simulink model "FullEKF_2007a"  (Simulink 6.6)
settings: Solver=FixedStepDiscrete  StartTime=0.0  StopTime=300  FixedStep=0.01  RelTol=1e-3
values from neighbouring files (symbols this model uses):
  initP = diag([1e-3 1e-3 1e-3 1e-6 1e-6 1e-6 1 1 1 5e-6 5e-6 5e-6 1e-8 1e-8 1e-8])    [FullEKF_init.m.m]
undefined symbols (not defined in the file or in its folder): DiscIntNeverNeededParam, gcbh, hwbcalib_subsystem
libraries: simulink x6, dspmtrx3 x4, dspinverses x1
(part 1 of 7)
settings Model: Creator=Markéta  LastModifiedBy=Markéta
settings OptimizationCC: InitFltsAndDblsToZero=off
settings DebuggingCC: StrictBusMsg=ErrorLevel1
settings HardwareCC: TargetHWDeviceType=32-bit Generic

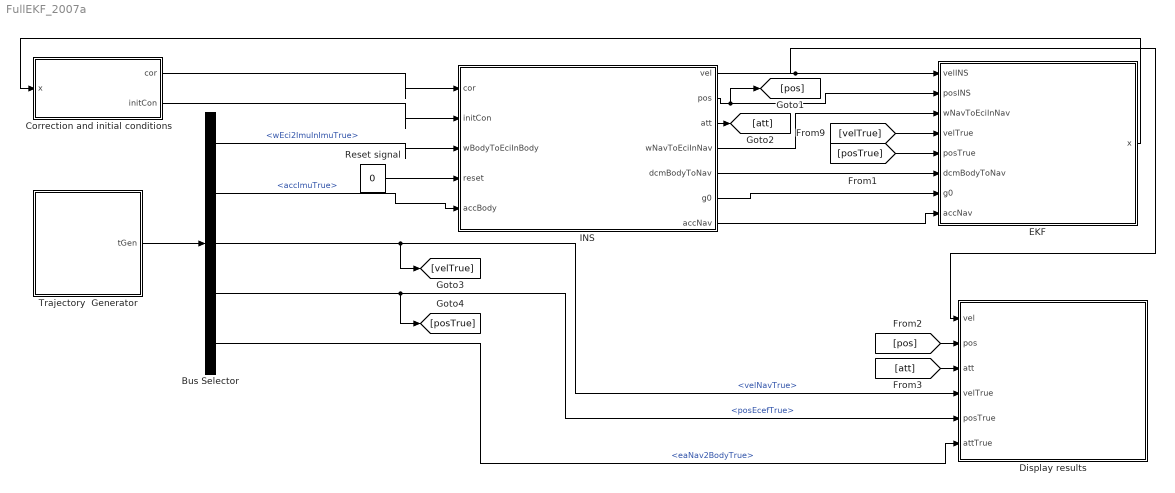
== system FullEKF_2007a ==
  Bus Selector : BusSelector  OutputSignals=state.wEci2ImuInImuTrue,state.accImuTrue,state.velNavTrue,state.posEcefTrue,state.eaNav2BodyTrue
  Correction and initial conditions : Subsystem
  Display results : Subsystem
  EKF : Subsystem
  INS : Subsystem
  Reset signal : Constant  Value=0  OutDataType=fixdt(1,16,0)  OutScaling=[]  SampleTime=0.01
  Trajectory  Generator : Subsystem
      settings: CopyFcn=|
      | if exist('gnlib_subsystem')
      |    gnlib_subsystem(gcbh, 'title')
      | end
      settings: NameChangeFcn=|
      | if exist('gnlib_subsystem')
      |    gnlib_subsystem(gcbh, 'title')
      | end
  wires:
  Trajectory  Generator/1(tGen) -> Bus Selector/1
  Bus Selector/2 -> INS/5(accBody)  "<accImuTrue>"
  Bus Selector/1 -> INS/3(wBodyToEciInBody)  "<wEci2ImuInImuTrue>"
  Correction and initial conditions/1(cor) -> INS/1(cor)
  Correction and initial conditions/2(initCon) -> INS/2(initCon)
  INS/1(vel) -> EKF/1(velINS), Display results/1(vel)
  INS/2(pos) -> EKF/2(posINS), [pos]
  Reset signal/1 -> INS/4(reset)
  EKF/1(x) -> Correction and initial conditions/1(x)
  INS/6(g0) -> EKF/7(g0)
  INS/4(wNavToEciInNav) -> EKF/3(wNavToEciInNav)
  INS/5(dcmBodyToNav) -> EKF/6(dcmBodyToNav)
  INS/7(accNav) -> EKF/8(accNav)
  Bus Selector/5 -> Display results/6(attTrue)  "<eaNav2BodyTrue>"
  Bus Selector/3 -> Display results/4(velTrue), [velTrue]  "<velNavTrue>"
  Bus Selector/4 -> Display results/5(posTrue), [posTrue]  "<posEcefTrue>"
  [posTrue] -> EKF/5(posTrue)
  [velTrue] -> EKF/4(velTrue)
  INS/3(att) -> [att]
  [att] -> Display results/3(att)
  [pos] -> Display results/2(pos)

== system FullEKF_2007a/Correction and initial conditions ==
  note: velInitCon
  note: posInitCon
  note: attInitCon
  note: corToAtt
  note: corToPos
  x : Inport  SampleTime=0.01  OutDataType=fixdt(1,16,0)  OutScaling=[]
  Bus Creator : BusCreator  Inputs=5
  Bus Creator1 : BusCreator  Inputs=3
  Demux : Demux  Outputs=5
  Demux2 : Demux  Outputs=3
  Gain{1..3,5} (4 alike) : Gain  ParameterDataType=fixdt(1,16,0)  ParameterScaling=[]  OutDataType=fixdt(1,16,0)  OutScaling=[]
  Gain4 : Gain  Gain=0  ParameterDataType=fixdt(1,16,0)  ParameterScaling=[]  OutDataType=fixdt(1,16,0)  OutScaling=[]
  accBias : Scope
      settings: TimeRange=50  YMin=-2.9e-014  YMax=-1.4e-014  SaveName=ScopeData4
  biasAcumulator1 : Subsystem
      settings: CopyFcn=|
      | if exist('gnlib_subsystem')
      |    gnlib_subsystem(gcbh, 'title')
      | end
      settings: NameChangeFcn=|
      | if exist('gnlib_subsystem')
      |    gnlib_subsystem(gcbh, 'title')
      | end
  biasAcumulator2 : Subsystem
      settings: CopyFcn=|
      | if exist('gnlib_subsystem')
      |    gnlib_subsystem(gcbh, 'title')
      | end
      settings: NameChangeFcn=|
      | if exist('gnlib_subsystem')
      |    gnlib_subsystem(gcbh, 'title')
      | end
  biasAcumulator3 : Subsystem
      settings: CopyFcn=|
      | if exist('gnlib_subsystem')
      |    gnlib_subsystem(gcbh, 'title')
      | end
      settings: NameChangeFcn=|
      | if exist('gnlib_subsystem')
      |    gnlib_subsystem(gcbh, 'title')
      | end
  biasAcumulator4 : Subsystem
      settings: CopyFcn=|
      | if exist('gnlib_subsystem')
      |    gnlib_subsystem(gcbh, 'title')
      | end
      settings: NameChangeFcn=|
      | if exist('gnlib_subsystem')
      |    gnlib_subsystem(gcbh, 'title')
      | end
  dcmInitCon : Constant  Value=[3.323433824319252e-14 -2.578151982846419e-07 1.570796798191198]  OutDataType=fixdt(1,16,0)  OutScaling=[]  SampleTime=0.01
  gyrBias : Scope  NumInputPorts=3
      settings: TimeRange=100  YMin=0.01825~0.0042~-0.014  YMax=0.02125~0.0059~-0.0075  SaveName=ScopeData5
  posInitCon : Constant  Value=[1.570796326794897; 0.7853981633974480; 0]  OutDataType=fixdt(1,16,0)  OutScaling=[]  SampleTime=0.01
  velInitCon : Constant  Value=[0 0 0]  OutDataType=fixdt(1,16,0)  OutScaling=[]  SampleTime=0.01
  cor : Outport  OutDataType=fixdt(1,16,0)  OutScaling=[]
  initCon : Outport  Port=2  OutDataType=fixdt(1,16,0)  OutScaling=[]
  wires:
  Bus Creator/1 -> cor/1
  velInitCon/1 -> Bus Creator1/1
  posInitCon/1 -> Bus Creator1/2
  dcmInitCon/1 -> Bus Creator1/3
  Bus Creator1/1 -> initCon/1
  x/1 -> Gain4/1
  Gain1/1 -> biasAcumulator2/1(dPos)
  Demux/1 -> Gain2/1
  biasAcumulator2/1(PosAcu) -> Bus Creator/2
  biasAcumulator4/1(accBiasAcu) -> Bus Creator/3
  Demux/2 -> Gain1/1
  Demux/3 -> Gain3/1
  Demux/4 -> biasAcumulator1/1(dAccBias)
  Demux/5 -> Gain5/1
  Gain3/1 -> biasAcumulator4/1(dAccBias)
  Gain2/1 -> Bus Creator/1
  Gain4/1 -> Demux/1
  Demux2/1 -> gyrBias/1
  Demux2/2 -> gyrBias/2
  Demux2/3 -> gyrBias/3
  biasAcumulator1/1(accBiasAcu) -> Bus Creator/4, accBias/1
  biasAcumulator3/1(accBiasAcu) -> Bus Creator/5, Demux2/1
  Gain5/1 -> biasAcumulator3/1(dAccBias)

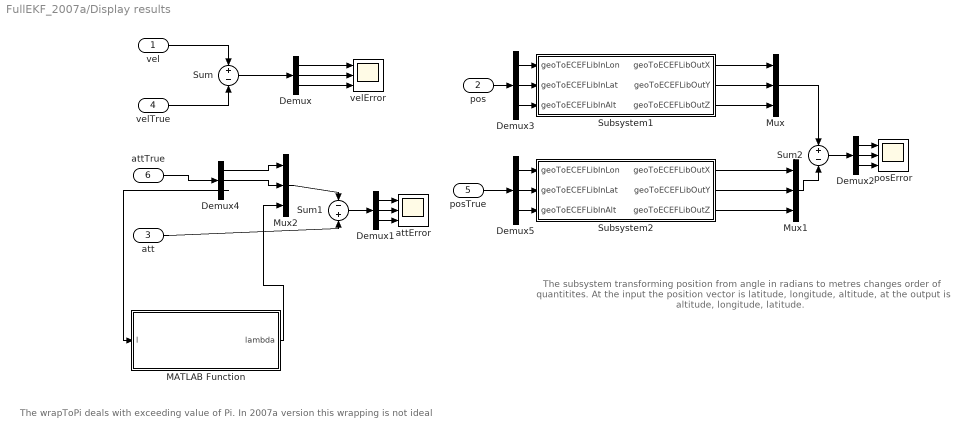
== system FullEKF_2007a/Display results ==
  note: The subsystem transforming position from angle in radians to metres changes
      | order of quantitites. At the input the position vector is latitude, longitude, altitude,
      | at the output is altitude, longitude, latitude.
  note: The wrapToPi deals with exceeding
      | value of Pi. In 2007a version this
      | wrapping is not ideal
  vel : Inport  PortDimensions=3  SampleTime=0.01  OutDataType=fixdt(1,16,0)  OutScaling=[]
  pos : Inport  Port=2  PortDimensions=3  SampleTime=0.01  OutDataType=fixdt(1,16,0)  OutScaling=[]
  att : Inport  Port=3  OutDataType=fixdt(1,16,0)  OutScaling=[]
  velTrue : Inport  Port=4  PortDimensions=3  SampleTime=0.01  OutDataType=fixdt(1,16,0)  OutScaling=[]
  posTrue : Inport  Port=5  PortDimensions=3  SampleTime=0.01  OutDataType=fixdt(1,16,0)  OutScaling=[]
  attTrue : Inport  Port=6  OutDataType=fixdt(1,16,0)  OutScaling=[]
  Demux{,1..5} (6 alike) : Demux  Outputs=3
  MATLAB Function : Stateflow chart  TreatAsAtomicUnit=on
  Mux : Mux  Inputs=3
  Mux1 : Mux  Inputs=3
  Mux2 : Mux  Inputs=3
  Subsystem1 : Subsystem
  Subsystem2 : Subsystem
  Sum : Sum  Inputs=+-  OutDataType=fixdt(1,16,0)  OutScaling=[]  SampleTime=0.01
  Sum1 : Sum  Inputs=-+  OutDataType=fixdt(1,16,0)  OutScaling=[]  SampleTime=0.01
  Sum2 : Sum  Inputs=+-  OutDataType=fixdt(1,16,0)  OutScaling=[]  SampleTime=0.01
  attError : Scope  NumInputPorts=3
      settings: YMin=-3e-007~-5e-007~6e-005  YMax=1e-006~9e-007~8.75e-005
  posError : Scope  NumInputPorts=3
      settings: TimeRange=100  YMin=-0.12~-0.325~-0.208  YMax=-0.103~-0.31~-0.197  SaveName=ScopeData2
  velError : Scope  NumInputPorts=3
      settings: TimeRange=300  YMin=-0.0075~-0.007~-0.007  YMax=0.0075~0.006~0.006
  wires:
  vel/1 -> Sum/1
  velTrue/1 -> Sum/2
  Sum2/1 -> Demux2/1
  Demux/1 -> velError/1
  Demux/2 -> velError/2
  Demux/3 -> velError/3
  Demux1/1 -> attError/1
  Demux1/2 -> attError/2
  Demux1/3 -> attError/3
  pos/1 -> Demux3/1
  posTrue/1 -> Demux5/1
  Mux/1 -> Sum2/1
  Mux1/1 -> Sum2/2
  Demux2/1 -> posError/1
  Demux2/2 -> posError/2
  Demux2/3 -> posError/3
  Demux3/1 -> Subsystem1/1(geoToECEFLibInLon)
  Demux3/2 -> Subsystem1/2(geoToECEFLibInLat)
  Demux3/3 -> Subsystem1/3(geoToECEFLibInAlt)
  Demux5/1 -> Subsystem2/1(geoToECEFLibInLon)
  Demux5/2 -> Subsystem2/2(geoToECEFLibInLat)
  Demux5/3 -> Subsystem2/3(geoToECEFLibInAlt)
  Subsystem1/2(geoToECEFLibOutY) -> Mux/2
  Subsystem2/2(geoToECEFLibOutY) -> Mux1/2
  Subsystem1/1(geoToECEFLibOutX) -> Mux/1
  Subsystem1/3(geoToECEFLibOutZ) -> Mux/3
  Subsystem2/3(geoToECEFLibOutZ) -> Mux1/3
  Subsystem2/1(geoToECEFLibOutX) -> Mux1/1
  Demux4/1 -> Mux2/1
  Demux4/2 -> Mux2/2
  Demux4/3 -> MATLAB Function/1(l)
  Mux2/1 -> Sum1/1
  MATLAB Function/1(lambda) -> Mux2/3
  attTrue/1 -> Demux4/1
  att/1 -> Sum1/2
  Sum1/1 -> Demux1/1
  Sum/1 -> Demux/1

== system FullEKF_2007a/EKF ==
  note: lon
  note: lat
  note: alt
  velINS : Inport  OutDataType=fixdt(1,16,0)  OutScaling=[]
  posINS : Inport  Port=2  OutDataType=fixdt(1,16,0)  OutScaling=[]
  wNavToEciInNav : Inport  Port=3  OutDataType=fixdt(1,16,0)  OutScaling=[]
  velTrue : Inport  Port=4  OutDataType=fixdt(1,16,0)  OutScaling=[]
  posTrue : Inport  Port=5  OutDataType=fixdt(1,16,0)  OutScaling=[]
  dcmBodyToNav : Inport  Port=6  PortDimensions=[3,3]  OutDataType=fixdt(1,16,0)  OutScaling=[]
  g0 : Inport  Port=7  OutDataType=fixdt(1,16,0)  OutScaling=[]
  accNav : Inport  Port=8  OutDataType=fixdt(1,16,0)  OutScaling=[]
  Demux : Demux  Outputs=3
  Demux1 : Demux  Outputs=3
  MATLAB Function : Stateflow chart  TreatAsAtomicUnit=on
  MeasureVector : Subsystem
  Terminator : Terminator
  Unit Delay : UnitDelay  X0=initP  SampleTime=-1
  Unit Delay1 : UnitDelay  X0=[0 0 0 0 0 0 0 0 0 0 0 0 0 0 0]  SampleTime=-1
  skewSymmetric : Subsystem  Tag=MBDLibrary v2007b.1  Description=|  TreatAsAtomicUnit=on
      | Skew Symmetric (MBDLibrary)                                                
      | Computes the Skew Symmetric Matrix Form of a vector.                       
      | output = [0  -omegaz omegay; omegaz 0 -omegax; -omegay omegax 0]           
      |                                                                            
      | %**************************************************************************
      | % HONEYWELL -CONFIDENTIAL: This copyrighted work and all information       
      | % are the property of Honeywell, contain trade secrets and may not,        
      | % in whole or in part, be used, duplicated, or disclosed for any purpose   
      | % without prior written permission of Honeywell.  All Rights Reserved.     
      | %                                                                          
      | % Notice                                                                   
      | % Freedom of Information Act (5 USC 552) and Disclosure of Confidential    
      | % Information Generally (18 USC 1905).  This material is being furnished   
      | % in confidence by Honeywell.  The information disclosed here falls        
      | % within exemption (b)(4) of 5 USC 552 and the prohibitions of             
      | % 18 USC 1905.                                                             
      | %                                                                          
      | % U.S. EXPORT CONTROL NOTICE:                                              
      | % This software is controlled in accordance with the United States Export  
      | % Administration Regulations (EAR).  This software has been classified as  
      | % EAR 99.  Diversion contrary to U.S. law is prohibited.                   
      | %**************************************************************************
      settings: OpenFcn=|
      | if exist('mbdlib_dialog')
      |    mbdlib_dialog(gcb,'open')
      | else
      |    open_system(gcb, 'mask')
      | end
      mask Type: Skew Symmetric (MBDLibrary)
      mask Description: Compute the Skew Symmetric Matrix Form of a Vector
      mask Help: The SKEW SYMMETRIC block computes the Skew Symmetric Matrix Form of a Vector
      mask Display:
      | plot([0.2 0.1 0.1 0.2], [0.95 0.95 0.05 0.05])
      | plot([0.8 0.9 0.9 0.8], [0.95 0.95 0.05 0.05])
      | text(0.5, 0.78, ' 0    -\omega_z   \omega_y', 'texmode', 'on')
      | text(0.5, 0.5, '  \omega_z   0   -\omega_x', 'texmode', 'on')
      | text(0.5, 0.22, '-\omega_y   \omega_x   0', 'texmode', 'on')
  skewSymmetric1 : Subsystem  Tag=MBDLibrary v2007b.1  Description=|  TreatAsAtomicUnit=on
      | Skew Symmetric (MBDLibrary)                                                
      | Computes the Skew Symmetric Matrix Form of a vector.                       
      | output = [0  -omegaz omegay; omegaz 0 -omegax; -omegay omegax 0]           
      |                                                                            
      | %**************************************************************************
      | % HONEYWELL -CONFIDENTIAL: This copyrighted work and all information       
      | % are the property of Honeywell, contain trade secrets and may not,        
      | % in whole or in part, be used, duplicated, or disclosed for any purpose   
      | % without prior written permission of Honeywell.  All Rights Reserved.     
      | %                                                                          
      | % Notice                                                                   
      | % Freedom of Information Act (5 USC 552) and Disclosure of Confidential    
      | % Information Generally (18 USC 1905).  This material is being furnished   
      | % in confidence by Honeywell.  The information disclosed here falls        
      | % within exemption (b)(4) of 5 USC 552 and the prohibitions of             
      | % 18 USC 1905.                                                             
      | %                                                                          
      | % U.S. EXPORT CONTROL NOTICE:                                              
      | % This software is controlled in accordance with the United States Export  
      | % Administration Regulations (EAR).  This software has been classified as  
      | % EAR 99.  Diversion contrary to U.S. law is prohibited.                   
      | %**************************************************************************
      settings: OpenFcn=|
      | if exist('mbdlib_dialog')
      |    mbdlib_dialog(gcb,'open')
      | else
      |    open_system(gcb, 'mask')
      | end
      mask Type: Skew Symmetric (MBDLibrary)
      mask Description: Compute the Skew Symmetric Matrix Form of a Vector
      mask Help: The SKEW SYMMETRIC block computes the Skew Symmetric Matrix Form of a Vector
      mask Display:
      | plot([0.2 0.1 0.1 0.2], [0.95 0.95 0.05 0.05])
      | plot([0.8 0.9 0.9 0.8], [0.95 0.95 0.05 0.05])
      | text(0.5, 0.78, ' 0    -\omega_z   \omega_y', 'texmode', 'on')
      | text(0.5, 0.5, '  \omega_z   0   -\omega_x', 'texmode', 'on')
      | text(0.5, 0.22, '-\omega_y   \omega_x   0', 'texmode', 'on')
  x : Outport  PortDimensions=[15,1]  OutDataType=fixdt(1,16,0)  OutScaling=[]
  wires:
  Unit Delay1/1 -> MATLAB Function/11(x_prev), x/1
  Demux1/1 -> MATLAB Function/6(velNorth)
  Demux1/2 -> MATLAB Function/7(velEast)
  Demux1/3 -> MATLAB Function/8(velDown)
  velTrue/1 -> MeasureVector/4(velTrue)
  wNavToEciInNav/1 -> skewSymmetric/1(skewLibIn)
  dcmBodyToNav/1 -> [dcmBodyToNav]
  posTrue/1 -> MeasureVector/3(posTrue)
  [g0] -> MATLAB Function/1(g0)
  g0/1 -> [g0]
  velINS/1 -> Demux1/1, MeasureVector/2(velINS)
  posINS/1 -> Demux/1, MeasureVector/1(posINS)
  [dcmBodyToNav] -> MATLAB Function/5(dcmBodyToNav)
  skewSymmetric/1(skewLibOut) -> MATLAB Function/2(wNavToEciInNav)
  MeasureVector/1(y) -> MATLAB Function/9(y)
  Unit Delay/1 -> MATLAB Function/12(P_prev)
  Demux/3 -> MATLAB Function/4(h)
  Demux/1 -> Terminator/1
  Demux/2 -> MATLAB Function/3(posLat)
  accNav/1 -> skewSymmetric1/1(skewLibIn)
  skewSymmetric1/1(skewLibOut) -> MATLAB Function/10(accNav)
  MATLAB Function/1(x) -> Unit Delay1/1
  MATLAB Function/2(P) -> Unit Delay/1

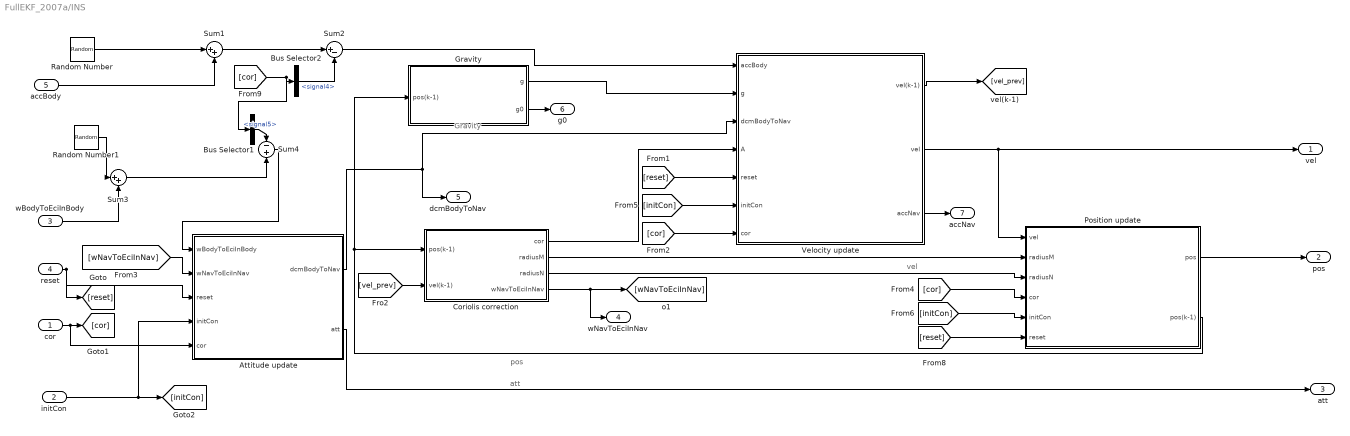
== system FullEKF_2007a/INS ==
  note: vel
  note: pos
  note: Gravity
  note: att
  cor : Inport  OutDataType=fixdt(1,16,0)  OutScaling=[]
  initCon : Inport  Port=2  OutDataType=fixdt(1,16,0)  OutScaling=[]
  wBodyToEciInBody : Inport  Port=3  PortDimensions=3  SampleTime=0.01  OutDataType=fixdt(1,16,0)  OutScaling=[]
  reset : Inport  Port=4  OutDataType=fixdt(1,16,0)  OutScaling=[]
  accBody : Inport  Port=5  PortDimensions=3  SampleTime=0.01  OutDataType=fixdt(1,16,0)  OutScaling=[]
  Attitude update : Subsystem
  Bus Selector1 : BusSelector  OutputSignals=signal5
  Bus Selector2 : BusSelector  OutputSignals=signal4
  Coriolis correction : Subsystem
  Gravity : Subsystem
  Position update : Subsystem
  Random Number : RandomNumber  Variance=0.0001  Seed=[55 45 60]  SampleTime=0.01
  Random Number1 : RandomNumber  Variance=4.3e-5  Seed=[55 45 60]  SampleTime=0.01
  Sum1 : Sum  Inputs=|++  OutDataType=fixdt(1,16,0)  OutScaling=[]
  Sum2 : Sum  Inputs=|+-  OutDataType=fixdt(1,16,0)  OutScaling=[]
  Sum3 : Sum  Inputs=|++  OutDataType=fixdt(1,16,0)  OutScaling=[]
  Sum4 : Sum  Inputs=-+  OutDataType=fixdt(1,16,0)  OutScaling=[]
  Velocity update : Subsystem
  vel : Outport  PortDimensions=3  SampleTime=0.01  OutDataType=fixdt(1,16,0)  OutScaling=[]
  pos : Outport  Port=2  PortDimensions=3  SampleTime=0.01  OutDataType=fixdt(1,16,0)  OutScaling=[]
  att : Outport  Port=3  PortDimensions=3  SampleTime=0.01  OutDataType=fixdt(1,16,0)  OutScaling=[]
  wNavToEciInNav : Outport  Port=4  PortDimensions=3  SampleTime=0.01  OutDataType=fixdt(1,16,0)  OutScaling=[]
  dcmBodyToNav : Outport  Port=5  PortDimensions=[3,3]  SampleTime=0.01  OutDataType=fixdt(1,16,0)  OutScaling=[]
  g0 : Outport  Port=6  PortDimensions=1  SampleTime=0.01  OutDataType=fixdt(1,16,0)  OutScaling=[]
  accNav : Outport  Port=7  PortDimensions=3  SampleTime=0.01  OutDataType=fixdt(1,16,0)  OutScaling=[]
  wires:
  Coriolis correction/2(radiusM) -> Position update/2(radiusM)
  Coriolis correction/3(radiusN) -> Position update/3(radiusN)
  Attitude update/1(dcmBodyToNav) -> dcmBodyToNav/1, Velocity update/3(dcmBodyToNav)
  reset/1 -> [reset], Attitude update/3(reset)
  [vel_prev] -> Coriolis correction/2(vel(k-1))
  Coriolis correction/4(wNavToEciInNav) -> [wNavToEciInNav], wNavToEciInNav/1
  Attitude update/2(att) -> att/1
  [wNavToEciInNav] -> Attitude update/2(wNavToEciInNav)
  Velocity update/1(vel(k-1)) -> [vel_prev]
  [cor] -> Position update/4(cor)
  initCon/1 -> [initCon], Attitude update/4(initCon)
  cor/1 -> [cor], Attitude update/5(cor)
  Position update/1(pos) -> pos/1
  [initCon] -> Position update/5(initCon)
  [reset] -> Position update/6(reset)
  Position update/2(pos(k-1)) -> Coriolis correction/1(pos(k-1)), Gravity/1(pos(k-1))
  Random Number/1 -> Sum1/1
  accBody/1 -> Sum1/2
  Gravity/2(g0) -> g0/1
  [cor] -> Velocity update/7(cor)
  [initCon] -> Velocity update/6(initCon)
  [reset] -> Velocity update/5(reset)
  Coriolis correction/1(cor) -> Velocity update/4(A)
  Gravity/1(g) -> Velocity update/2(g)
  Velocity update/3(accNav) -> accNav/1
  Velocity update/2(vel) -> vel/1, Position update/1(vel)
  [cor] -> Bus Selector2/1, Bus Selector1/1
  Bus Selector2/1 -> Sum2/2  "<signal4>"
  Sum1/1 -> Sum2/1
  Sum2/1 -> Velocity update/1(accBody)
  Random Number1/1 -> Sum3/1
  wBodyToEciInBody/1 -> Sum3/2
  Bus Selector1/1 -> Sum4/1  "<signal5>"
  Sum4/1 -> Attitude update/1(wBodyToEciInBody)
  Sum3/1 -> Sum4/2

== system FullEKF_2007a/Trajectory  Generator ==
  note: Notes:
      | 1. Generating input trajectory true values for sensor models
  note: Trajectory
      | Generator
  note: Acc and Gyro IMU inputs
  Bus Creator1 : BusCreator  Inputs=2
  Signals Conversions dtgen : Subsystem
      settings: CopyFcn=|
      | if exist('gnlib_subsystem')
      |    gnlib_subsystem(gcbh, 'title')
      | end
      settings: NameChangeFcn=|
      | if exist('gnlib_subsystem')
      |    gnlib_subsystem(gcbh, 'title')
      | end
  Signals Conversions trmodel : Subsystem
      settings: CopyFcn=|
      | if exist('gnlib_subsystem')
      |    gnlib_subsystem(gcbh, 'title')
      | end
      settings: NameChangeFcn=|
      | if exist('gnlib_subsystem')
      |    gnlib_subsystem(gcbh, 'title')
      | end
  dtgen : FromWorkspace  VariableName=dtgen  SampleTime=0.01  OutputAfterFinalValue=Setting to zero
  trmodel : FromWorkspace  VariableName=trmodel  SampleTime=0  OutputAfterFinalValue=Setting to zero
  tGen : Outport  OutDataType=fixdt(1,16,0)  OutScaling=[]
  wires:
  dtgen/1 -> Signals Conversions trmodel/1(dtgen)
  trmodel/1 -> Signals Conversions dtgen/1(trmodel)
  Signals Conversions dtgen/1(state) -> Bus Creator1/1  "state"
  Signals Conversions trmodel/1(imu) -> Bus Creator1/2  "imu"
  Bus Creator1/1 -> tGen/1

== system FullEKF_2007a/Correction and initial conditions/biasAcumulator1 ==
  dAccBias : Inport  OutDataType=fixdt(1,16,0)  OutScaling=[]
  1/2 : Gain  Orientation=left  ParameterDataType=fixdt(1,16,0)  ParameterScaling=[]  OutDataType=fixdt(1,16,0)  OutScaling=[]  SaturateOnIntegerOverflow=on
  Sum : Sum  Inputs=|++  OutDataType=fixdt(1,16,0)  OutScaling=[]
  Unit Delay5 : UnitDelay  Orientation=left  SampleTime=-1
  accBiasAcu : Outport  OutDataType=fixdt(1,16,0)  OutScaling=[]
  wires:
  Sum/1 -> accBiasAcu/1, 1/2/1
  dAccBias/1 -> Sum/1
  1/2/1 -> Unit Delay5/1
  Unit Delay5/1 -> Sum/2

== system FullEKF_2007a/Correction and initial conditions/biasAcumulator2 ==
  dPos : Inport  OutDataType=fixdt(1,16,0)  OutScaling=[]
  1/2 : Gain  Orientation=left  ParameterDataType=fixdt(1,16,0)  ParameterScaling=[]  OutDataType=fixdt(1,16,0)  OutScaling=[]  SaturateOnIntegerOverflow=on
  Sum : Sum  Inputs=|++  OutDataType=fixdt(1,16,0)  OutScaling=[]
  Unit Delay5 : UnitDelay  Orientation=left  SampleTime=-1
  PosAcu : Outport  OutDataType=fixdt(1,16,0)  OutScaling=[]
  wires:
  Sum/1 -> PosAcu/1, 1/2/1
  dPos/1 -> Sum/1
  1/2/1 -> Unit Delay5/1
  Unit Delay5/1 -> Sum/2

== system FullEKF_2007a/Correction and initial conditions/biasAcumulator3 ==
  dAccBias : Inport  OutDataType=fixdt(1,16,0)  OutScaling=[]
  1/2 : Gain  Orientation=left  ParameterDataType=fixdt(1,16,0)  ParameterScaling=[]  OutDataType=fixdt(1,16,0)  OutScaling=[]  SaturateOnIntegerOverflow=on
  Sum : Sum  Inputs=|++  OutDataType=fixdt(1,16,0)  OutScaling=[]
  Unit Delay5 : UnitDelay  Orientation=left  SampleTime=-1
  accBiasAcu : Outport  OutDataType=fixdt(1,16,0)  OutScaling=[]
  wires:
  Sum/1 -> accBiasAcu/1, 1/2/1
  dAccBias/1 -> Sum/1
  1/2/1 -> Unit Delay5/1
  Unit Delay5/1 -> Sum/2

== system FullEKF_2007a/Correction and initial conditions/biasAcumulator4 ==
  dAccBias : Inport  OutDataType=fixdt(1,16,0)  OutScaling=[]
  1/2 : Gain  Orientation=left  ParameterDataType=fixdt(1,16,0)  ParameterScaling=[]  OutDataType=fixdt(1,16,0)  OutScaling=[]  SaturateOnIntegerOverflow=on
  Sum : Sum  Inputs=|++  OutDataType=fixdt(1,16,0)  OutScaling=[]
  Unit Delay5 : UnitDelay  Orientation=left  SampleTime=-1
  accBiasAcu : Outport  OutDataType=fixdt(1,16,0)  OutScaling=[]
  wires:
  Sum/1 -> accBiasAcu/1, 1/2/1
  dAccBias/1 -> Sum/1
  1/2/1 -> Unit Delay5/1
  Unit Delay5/1 -> Sum/2

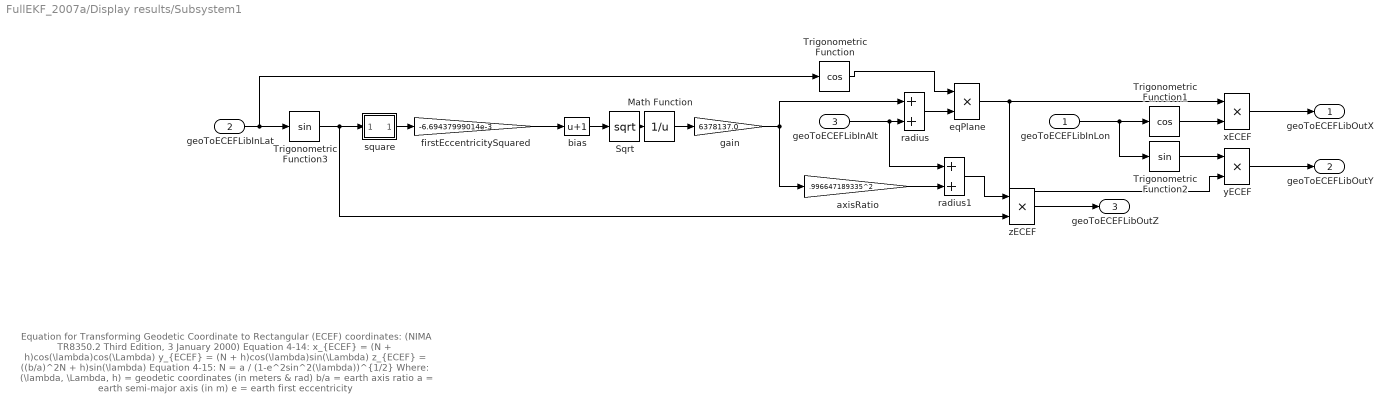
== system FullEKF_2007a/Display results/Subsystem1 ==
  note: Equation for Transforming Geodetic Coordinate
      | to Rectangular (ECEF) coordinates:
      | (NIMA TR8350.2 Third Edition, 3 January 2000)
      |
      | Equation 4-14:
      | x_{ECEF} = (N + h)cos(\lambda)cos(\Lambda)
      | y_{ECEF} = (N + h)cos(\lambda)sin(\Lambda)
      | z_{ECEF} = ((b/a)^2N + h)sin(\lambda)
      |
      | Equation 4-15:
      | N = a / (1-e^2sin^2(\lambda))^{1/2}
      |
      | Where:
      | (\lambda, \Lambda, h) = geodetic coordinates (in meters & rad)
      | b/a = earth axis ratio
      | a = earth semi-major axis (in m)
      | e = earth first eccentricity
  geoToECEFLibInLon : Inport  OutDataType=fixdt(1,16,0)  OutScaling=[]
  geoToECEFLibInLat : Inport  Port=2  OutDataType=fixdt(1,16,0)  OutScaling=[]
  geoToECEFLibInAlt : Inport  Port=3  OutDataType=fixdt(1,16,0)  OutScaling=[]
  Math Function : Math  Operator=reciprocal  OutDataType=fixdt(1,16,0)  OutScaling=[]  SaturateOnIntegerOverflow=on
  Sqrt : Math  Operator=sqrt  OutDataType=fixdt(1,16,0)  OutScaling=[]  SaturateOnIntegerOverflow=on
  Trigonometric Function : Trigonometry  Operator=cos
  Trigonometric Function1 : Trigonometry  Operator=cos
  Trigonometric Function2 : Trigonometry
  Trigonometric Function3 : Trigonometry
  axisRatio : Gain  Tag=MBDLibrary v2007b.1  Gain=.996647189335^2  ParameterDataType=fixdt(1,16,0)  ParameterScaling=[]  OutDataType=fixdt(1,16,0)  OutScaling=[]  RndMeth=Zero  mask(Gain (MBDLibrary)){gain_mbdlib=.996647189335^2}
      mask prompts: gain_mbdlib "Gain"
      mask help: Multiplies the input by the gain.
      settings: OpenFcn=|
      | if exist('mbdlib_dialog')
      |    mbdlib_dialog(gcb,'open')
      | else
      |    open_system(gcb, 'mask')
      | end
      mask Help: The GAIN block multiplies the input by the gain value.  This block may accept any data types other than boolean.  The user must take care to not use a non-integer gain for int32/uint32 inputs.
      mask Display: disp([get_param(gcb, 'Gain') 'x'])
  bias : Bias  Tag=MBDLibrary v2007b.1  Bias=1  mask(Bias (MBDLibrary)){Bias_mbdlib=1}
      mask prompts: Bias_mbdlib "Bias"
      mask help: Add bias to input.
      settings: OpenFcn=|
      | if exist('mbdlib_dialog')
      |    mbdlib_dialog(gcb,'open')
      | else
      |    open_system(gcb, 'mask')
      | end
      settings: CloseFcn=|
      | if exist('mbdlib_bias')
      |    mbdlib_bias(gcb)
      | end
      mask Help: The BIAS block outputs the summation of an input with a specified constant.
      mask Display: disp(['x+1'])
  eqPlane : Product  Tag=MBDLibrary v2007b.1  OutDataType=fixdt(1,16,0)  OutScaling=[]  RndMeth=Zero  InputSameDT=on  mask(Product (MBDLibrary)){Inputs_mbdlib=2}
      mask prompts: Inputs_mbdlib "Number of Inputs"
      mask help: Multiplies inputs.
      settings: OpenFcn=|
      | if exist('mbdlib_dialog')
      |    mbdlib_dialog(gcb,'open')
      | else
      |    open_system(gcb, 'mask')
      | end
      mask Help: The PRODUCT block is used to multiply inputs.
  firstEccentricitySquared : Gain  Tag=MBDLibrary v2007b.1  Gain=-6.69437999014e-3  ParameterDataType=fixdt(1,16,0)  ParameterScaling=[]  OutDataType=fixdt(1,16,0)  OutScaling=[]  RndMeth=Zero  mask(Gain (MBDLibrary)){gain_mbdlib=-6.69437999014e-3}
      mask prompts: gain_mbdlib "Gain"
      mask help: Multiplies the input by the gain.
      settings: OpenFcn=|
      | if exist('mbdlib_dialog')
      |    mbdlib_dialog(gcb,'open')
      | else
      |    open_system(gcb, 'mask')
      | end
      mask Help: The GAIN block multiplies the input by the gain value.  This block may accept any data types other than boolean.  The user must take care to not use a non-integer gain for int32/uint32 inputs.
      mask Display: disp([get_param(gcb, 'Gain') 'x'])
  gain : Gain  Tag=MBDLibrary v2007b.1  Gain=6378137.0  ParameterDataType=fixdt(1,16,0)  ParameterScaling=[]  OutDataType=fixdt(1,16,0)  OutScaling=[]  RndMeth=Zero  mask(Gain (MBDLibrary)){gain_mbdlib=6378137.0}
      mask prompts: gain_mbdlib "Gain"
      mask help: Multiplies the input by the gain.
      settings: OpenFcn=|
      | if exist('mbdlib_dialog')
      |    mbdlib_dialog(gcb,'open')
      | else
      |    open_system(gcb, 'mask')
      | end
      mask Help: The GAIN block multiplies the input by the gain value.  This block may accept any data types other than boolean.  The user must take care to not use a non-integer gain for int32/uint32 inputs.
      mask Display: disp([get_param(gcb, 'Gain') 'x'])
  radius : Sum  Tag=MBDLibrary v2007b.1  OutDataType=fixdt(1,16,0)  OutScaling=[]  RndMeth=Zero  InputSameDT=on  mask(Sum (MBDLibrary)){inputs_mbdlib=++}
      mask prompts: inputs_mbdlib "List of signs"
      mask help: Adds values together.
      settings: OpenFcn=|
      | if exist('mbdlib_dialog')
      |    mbdlib_dialog(gcb,'open')
      | else
      |    open_system(gcb, 'mask')
      | end
      mask Help:
      | The SUM block is used to add or subtract  inputs.
      | The inputs may be specified as:
      |   (a) + or - for each port (i.e. ++-+)
      |   (b) An integer to indicate the number of ports to add
      | Note that the number of ports input to this block must be between 1 and 25.
      | When only 1 inport is selected, the block computes the summation of vector input elements and outputs a scalar.
  radius1 : Sum  Tag=MBDLibrary v2007b.1  OutDataType=fixdt(1,16,0)  OutScaling=[]  RndMeth=Zero  InputSameDT=on  mask(Sum (MBDLibrary)){inputs_mbdlib=++}
      mask prompts: inputs_mbdlib "List of signs"
      mask help: Adds values together.
      settings: OpenFcn=|
      | if exist('mbdlib_dialog')
      |    mbdlib_dialog(gcb,'open')
      | else
      |    open_system(gcb, 'mask')
      | end
      mask Help:
      | The SUM block is used to add or subtract  inputs.
      | The inputs may be specified as:
      |   (a) + or - for each port (i.e. ++-+)
      |   (b) An integer to indicate the number of ports to add
      | Note that the number of ports input to this block must be between 1 and 25.
      | When only 1 inport is selected, the block computes the summation of vector input elements and outputs a scalar.
  square : Subsystem  Tag=MBDLibrary v2007b.1
      settings: OpenFcn=|
      | if exist('mbdlib_dialog')
      |    mbdlib_dialog(gcb,'open')
      | else
      |    open_system(gcb, 'mask')
      | end
      mask Type: Square (MBDLibrary)
      mask Description: Squares the input.
      mask Help: The SQAURE block outputs the square of the input value.
      mask Display: disp('x^2', 'texmode', 'on')
  xECEF : Product  Tag=MBDLibrary v2007b.1  OutDataType=fixdt(1,16,0)  OutScaling=[]  RndMeth=Zero  InputSameDT=on  mask(Product (MBDLibrary)){Inputs_mbdlib=2}
      mask prompts: Inputs_mbdlib "Number of Inputs"
      mask help: Multiplies inputs.
      settings: OpenFcn=|
      | if exist('mbdlib_dialog')
      |    mbdlib_dialog(gcb,'open')
      | else
      |    open_system(gcb, 'mask')
      | end
      mask Help: The PRODUCT block is used to multiply inputs.
  yECEF : Product  Tag=MBDLibrary v2007b.1  OutDataType=fixdt(1,16,0)  OutScaling=[]  RndMeth=Zero  InputSameDT=on  mask(Product (MBDLibrary)){Inputs_mbdlib=2}
      mask prompts: Inputs_mbdlib "Number of Inputs"
      mask help: Multiplies inputs.
      settings: OpenFcn=|
      | if exist('mbdlib_dialog')
      |    mbdlib_dialog(gcb,'open')
      | else
      |    open_system(gcb, 'mask')
      | end
      mask Help: The PRODUCT block is used to multiply inputs.
  zECEF : Product  Tag=MBDLibrary v2007b.1  OutDataType=fixdt(1,16,0)  OutScaling=[]  RndMeth=Zero  InputSameDT=on  mask(Product (MBDLibrary)){Inputs_mbdlib=2}
      mask prompts: Inputs_mbdlib "Number of Inputs"
      mask help: Multiplies inputs.
      settings: OpenFcn=|
      | if exist('mbdlib_dialog')
      |    mbdlib_dialog(gcb,'open')
      | else
      |    open_system(gcb, 'mask')
      | end
      mask Help: The PRODUCT block is used to multiply inputs.
  geoToECEFLibOutX : Outport  OutDataType=fixdt(1,16,0)  OutScaling=[]
  geoToECEFLibOutY : Outport  Port=2  OutDataType=fixdt(1,16,0)  OutScaling=[]
  geoToECEFLibOutZ : Outport  Port=3  OutDataType=fixdt(1,16,0)  OutScaling=[]
  wires:
  Trigonometric Function3/1 -> zECEF/2, square/1(squareLibIn)
  zECEF/1 -> geoToECEFLibOutZ/1
  yECEF/1 -> geoToECEFLibOutY/1
  xECEF/1 -> geoToECEFLibOutX/1
  radius1/1 -> zECEF/1
  eqPlane/1 -> yECEF/2, xECEF/1
  Trigonometric Function2/1 -> yECEF/1
  geoToECEFLibInLon/1 -> Trigonometric Function1/1, Trigonometric Function2/1
  axisRatio/1 -> radius1/2
  geoToECEFLibInAlt/1 -> radius1/1, radius/2
  gain/1 -> axisRatio/1, radius/1
  Trigonometric Function/1 -> eqPlane/1
  Trigonometric Function1/1 -> xECEF/2
  radius/1 -> eqPlane/2
  bias/1 -> Sqrt/1
  firstEccentricitySquared/1 -> bias/1
  square/1(squareLibOut) -> firstEccentricitySquared/1
  geoToECEFLibInLat/1 -> Trigonometric Function/1, Trigonometric Function3/1
  Sqrt/1 -> Math Function/1
  Math Function/1 -> gain/1

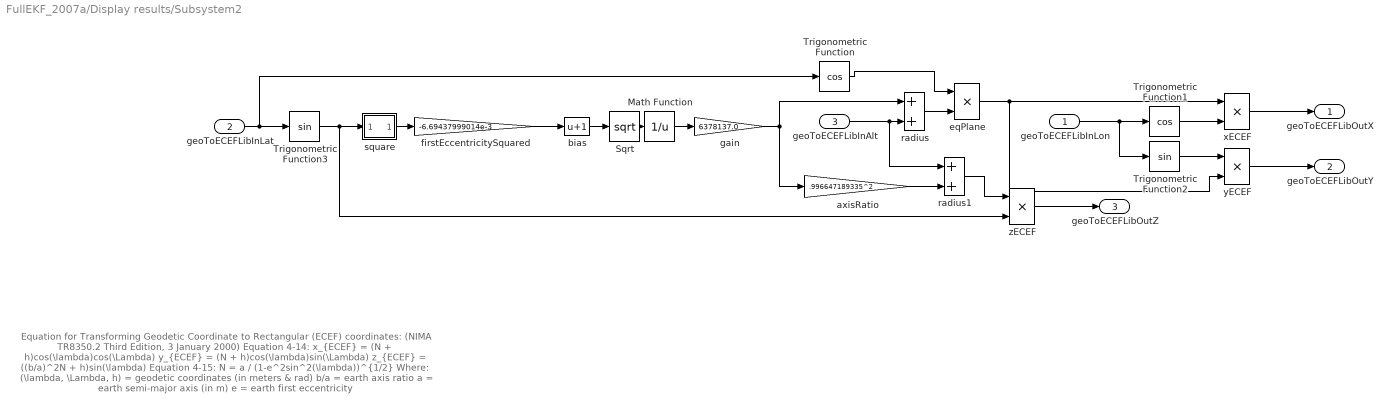
== system FullEKF_2007a/Display results/Subsystem2 ==
  note: Equation for Transforming Geodetic Coordinate
      | to Rectangular (ECEF) coordinates:
      | (NIMA TR8350.2 Third Edition, 3 January 2000)
      |
      | Equation 4-14:
      | x_{ECEF} = (N + h)cos(\lambda)cos(\Lambda)
      | y_{ECEF} = (N + h)cos(\lambda)sin(\Lambda)
      | z_{ECEF} = ((b/a)^2N + h)sin(\lambda)
      |
      | Equation 4-15:
      | N = a / (1-e^2sin^2(\lambda))^{1/2}
      |
      | Where:
      | (\lambda, \Lambda, h) = geodetic coordinates (in meters & rad)
      | b/a = earth axis ratio
      | a = earth semi-major axis (in m)
      | e = earth first eccentricity
  geoToECEFLibInLon : Inport  OutDataType=fixdt(1,16,0)  OutScaling=[]
  geoToECEFLibInLat : Inport  Port=2  OutDataType=fixdt(1,16,0)  OutScaling=[]
  geoToECEFLibInAlt : Inport  Port=3  OutDataType=fixdt(1,16,0)  OutScaling=[]
  Math Function : Math  Operator=reciprocal  OutDataType=fixdt(1,16,0)  OutScaling=[]  SaturateOnIntegerOverflow=on
  Sqrt : Math  Operator=sqrt  OutDataType=fixdt(1,16,0)  OutScaling=[]  SaturateOnIntegerOverflow=on
  Trigonometric Function : Trigonometry  Operator=cos
  Trigonometric Function1 : Trigonometry  Operator=cos
  Trigonometric Function2 : Trigonometry
  Trigonometric Function3 : Trigonometry
  axisRatio : Gain  Tag=MBDLibrary v2007b.1  Gain=.996647189335^2  ParameterDataType=fixdt(1,16,0)  ParameterScaling=[]  OutDataType=fixdt(1,16,0)  OutScaling=[]  RndMeth=Zero  mask(Gain (MBDLibrary)){gain_mbdlib=.996647189335^2}
      mask prompts: gain_mbdlib "Gain"
      mask help: Multiplies the input by the gain.
      settings: OpenFcn=|
      | if exist('mbdlib_dialog')
      |    mbdlib_dialog(gcb,'open')
      | else
      |    open_system(gcb, 'mask')
      | end
      mask Help: The GAIN block multiplies the input by the gain value.  This block may accept any data types other than boolean.  The user must take care to not use a non-integer gain for int32/uint32 inputs.
      mask Display: disp([get_param(gcb, 'Gain') 'x'])
  bias : Bias  Tag=MBDLibrary v2007b.1  Bias=1  mask(Bias (MBDLibrary)){Bias_mbdlib=1}
      mask prompts: Bias_mbdlib "Bias"
      mask help: Add bias to input.
      settings: OpenFcn=|
      | if exist('mbdlib_dialog')
      |    mbdlib_dialog(gcb,'open')
      | else
      |    open_system(gcb, 'mask')
      | end
      settings: CloseFcn=|
      | if exist('mbdlib_bias')
      |    mbdlib_bias(gcb)
      | end
      mask Help: The BIAS block outputs the summation of an input with a specified constant.
      mask Display: disp(['x+1'])
  eqPlane : Product  Tag=MBDLibrary v2007b.1  OutDataType=fixdt(1,16,0)  OutScaling=[]  RndMeth=Zero  InputSameDT=on  mask(Product (MBDLibrary)){Inputs_mbdlib=2}
      mask prompts: Inputs_mbdlib "Number of Inputs"
      mask help: Multiplies inputs.
      settings: OpenFcn=|
      | if exist('mbdlib_dialog')
      |    mbdlib_dialog(gcb,'open')
      | else
      |    open_system(gcb, 'mask')
      | end
      mask Help: The PRODUCT block is used to multiply inputs.
  firstEccentricitySquared : Gain  Tag=MBDLibrary v2007b.1  Gain=-6.69437999014e-3  ParameterDataType=fixdt(1,16,0)  ParameterScaling=[]  OutDataType=fixdt(1,16,0)  OutScaling=[]  RndMeth=Zero  mask(Gain (MBDLibrary)){gain_mbdlib=-6.69437999014e-3}
      mask prompts: gain_mbdlib "Gain"
      mask help: Multiplies the input by the gain.
      settings: OpenFcn=|
      | if exist('mbdlib_dialog')
      |    mbdlib_dialog(gcb,'open')
      | else
      |    open_system(gcb, 'mask')
      | end
      mask Help: The GAIN block multiplies the input by the gain value.  This block may accept any data types other than boolean.  The user must take care to not use a non-integer gain for int32/uint32 inputs.
      mask Display: disp([get_param(gcb, 'Gain') 'x'])
  gain : Gain  Tag=MBDLibrary v2007b.1  Gain=6378137.0  ParameterDataType=fixdt(1,16,0)  ParameterScaling=[]  OutDataType=fixdt(1,16,0)  OutScaling=[]  RndMeth=Zero  mask(Gain (MBDLibrary)){gain_mbdlib=6378137.0}
      mask prompts: gain_mbdlib "Gain"
      mask help: Multiplies the input by the gain.
      settings: OpenFcn=|
      | if exist('mbdlib_dialog')
      |    mbdlib_dialog(gcb,'open')
      | else
      |    open_system(gcb, 'mask')
      | end
      mask Help: The GAIN block multiplies the input by the gain value.  This block may accept any data types other than boolean.  The user must take care to not use a non-integer gain for int32/uint32 inputs.
      mask Display: disp([get_param(gcb, 'Gain') 'x'])
  radius : Sum  Tag=MBDLibrary v2007b.1  OutDataType=fixdt(1,16,0)  OutScaling=[]  RndMeth=Zero  InputSameDT=on  mask(Sum (MBDLibrary)){inputs_mbdlib=++}
      mask prompts: inputs_mbdlib "List of signs"
      mask help: Adds values together.
      settings: OpenFcn=|
      | if exist('mbdlib_dialog')
      |    mbdlib_dialog(gcb,'open')
      | else
      |    open_system(gcb, 'mask')
      | end
      mask Help:
      | The SUM block is used to add or subtract  inputs.
      | The inputs may be specified as:
      |   (a) + or - for each port (i.e. ++-+)
      |   (b) An integer to indicate the number of ports to add
      | Note that the number of ports input to this block must be between 1 and 25.
      | When only 1 inport is selected, the block computes the summation of vector input elements and outputs a scalar.
  radius1 : Sum  Tag=MBDLibrary v2007b.1  OutDataType=fixdt(1,16,0)  OutScaling=[]  RndMeth=Zero  InputSameDT=on  mask(Sum (MBDLibrary)){inputs_mbdlib=++}
      mask prompts: inputs_mbdlib "List of signs"
      mask help: Adds values together.
      settings: OpenFcn=|
      | if exist('mbdlib_dialog')
      |    mbdlib_dialog(gcb,'open')
      | else
      |    open_system(gcb, 'mask')
      | end
      mask Help:
      | The SUM block is used to add or subtract  inputs.
      | The inputs may be specified as:
      |   (a) + or - for each port (i.e. ++-+)
      |   (b) An integer to indicate the number of ports to add
      | Note that the number of ports input to this block must be between 1 and 25.
      | When only 1 inport is selected, the block computes the summation of vector input elements and outputs a scalar.
  square : Subsystem  Tag=MBDLibrary v2007b.1
      settings: OpenFcn=|
      | if exist('mbdlib_dialog')
      |    mbdlib_dialog(gcb,'open')
      | else
      |    open_system(gcb, 'mask')
      | end
      mask Type: Square (MBDLibrary)
      mask Description: Squares the input.
      mask Help: The SQAURE block outputs the square of the input value.
      mask Display: disp('x^2', 'texmode', 'on')
  xECEF : Product  Tag=MBDLibrary v2007b.1  OutDataType=fixdt(1,16,0)  OutScaling=[]  RndMeth=Zero  InputSameDT=on  mask(Product (MBDLibrary)){Inputs_mbdlib=2}
      mask prompts: Inputs_mbdlib "Number of Inputs"
      mask help: Multiplies inputs.
      settings: OpenFcn=|
      | if exist('mbdlib_dialog')
      |    mbdlib_dialog(gcb,'open')
      | else
      |    open_system(gcb, 'mask')
      | end
      mask Help: The PRODUCT block is used to multiply inputs.
  yECEF : Product  Tag=MBDLibrary v2007b.1  OutDataType=fixdt(1,16,0)  OutScaling=[]  RndMeth=Zero  InputSameDT=on  mask(Product (MBDLibrary)){Inputs_mbdlib=2}
      mask prompts: Inputs_mbdlib "Number of Inputs"
      mask help: Multiplies inputs.
      settings: OpenFcn=|
      | if exist('mbdlib_dialog')
      |    mbdlib_dialog(gcb,'open')
      | else
      |    open_system(gcb, 'mask')
      | end
      mask Help: The PRODUCT block is used to multiply inputs.
  zECEF : Product  Tag=MBDLibrary v2007b.1  OutDataType=fixdt(1,16,0)  OutScaling=[]  RndMeth=Zero  InputSameDT=on  mask(Product (MBDLibrary)){Inputs_mbdlib=2}
      mask prompts: Inputs_mbdlib "Number of Inputs"
      mask help: Multiplies inputs.
      settings: OpenFcn=|
      | if exist('mbdlib_dialog')
      |    mbdlib_dialog(gcb,'open')
      | else
      |    open_system(gcb, 'mask')
      | end
      mask Help: The PRODUCT block is used to multiply inputs.
  geoToECEFLibOutX : Outport  OutDataType=fixdt(1,16,0)  OutScaling=[]
  geoToECEFLibOutY : Outport  Port=2  OutDataType=fixdt(1,16,0)  OutScaling=[]
  geoToECEFLibOutZ : Outport  Port=3  OutDataType=fixdt(1,16,0)  OutScaling=[]
  wires:
  Trigonometric Function3/1 -> zECEF/2, square/1(squareLibIn)
  zECEF/1 -> geoToECEFLibOutZ/1
  yECEF/1 -> geoToECEFLibOutY/1
  xECEF/1 -> geoToECEFLibOutX/1
  radius1/1 -> zECEF/1
  eqPlane/1 -> yECEF/2, xECEF/1
  Trigonometric Function2/1 -> yECEF/1
  geoToECEFLibInLon/1 -> Trigonometric Function1/1, Trigonometric Function2/1
  axisRatio/1 -> radius1/2
  geoToECEFLibInAlt/1 -> radius1/1, radius/2
  gain/1 -> axisRatio/1, radius/1
  Trigonometric Function/1 -> eqPlane/1
  Trigonometric Function1/1 -> xECEF/2
  radius/1 -> eqPlane/2
  bias/1 -> Sqrt/1
  firstEccentricitySquared/1 -> bias/1
  square/1(squareLibOut) -> firstEccentricitySquared/1
  geoToECEFLibInLat/1 -> Trigonometric Function/1, Trigonometric Function3/1
  Sqrt/1 -> Math Function/1
  Math Function/1 -> gain/1

== system FullEKF_2007a/EKF/MeasureVector ==
  posINS : Inport  OutDataType=fixdt(1,16,0)  OutScaling=[]
  velINS : Inport  Port=2  OutDataType=fixdt(1,16,0)  OutScaling=[]
  posTrue : Inport  Port=3  OutDataType=fixdt(1,16,0)  OutScaling=[]
  velTrue : Inport  Port=4  OutDataType=fixdt(1,16,0)  OutScaling=[]
  GPS : Subsystem
  MATLAB Function : Stateflow chart  TreatAsAtomicUnit=on
  y : Outport  OutDataType=fixdt(1,16,0)  OutScaling=[]
  wires:
  posTrue/1 -> GPS/1(posTrue)
  velTrue/1 -> GPS/2(velTrue)
  MATLAB Function/1(y) -> y/1
  posINS/1 -> MATLAB Function/1(posIns)
  GPS/2(velGps) -> MATLAB Function/4(velGps)
  velINS/1 -> MATLAB Function/3(velIns)
  GPS/1(posGps) -> MATLAB Function/2(posGps)

== system FullEKF_2007a/EKF/skewSymmetric ==
  skewLibIn : Inport  OutDataType=fixdt(1,16,0)  OutScaling=[]
  column1 : Selector  Tag=MBDLibrary v2007b.1  IndexOptions=Index vector (dialog)  Indices=[7 3 5]  OutputSizes=1  InputPortWidth=7  mask(Mux Selector (MBDLibrary)){InputPortWidth_mbdlib=7, Indices_mbdlib=[7 3 5]}
      mask prompts: InputPortWidth_mbdlib "Input Port Width"; Indices_mbdlib "Output Indices"
      mask help: Changes the order of the inputs.
      settings: OpenFcn=|
      | if exist('mbdlib_dialog')
      |    mbdlib_dialog(gcb,'open')
      | else
      |    open_system(gcb, 'mask')
      | end
      settings: CloseFcn=|
      | if exist('mbdlib_selector')
      |    mbdlib_selector(gcb)
      | end
      mask Help: The SELECTOR block is a MULTIPLEXED SELECTOR block, used to change the input/output order of a multiplexed data stream.
      mask Display:
      | port_label('input', 1,'[7]')
      | text(1.0,0.83333,'7', 'horizontalAlignment', 'right')
      | text(1.0,0.5,'3', 'horizontalAlignment', 'right')
      | text(1.0,0.16667,'5', 'horizontalAlignment', 'right')
  column2 : Selector  Tag=MBDLibrary v2007b.1  IndexOptions=Index vector (dialog)  Indices=[6 7 1]  OutputSizes=1  InputPortWidth=7  mask(Mux Selector (MBDLibrary)){InputPortWidth_mbdlib=7, Indices_mbdlib=[6 7 1]}
      mask prompts: InputPortWidth_mbdlib "Input Port Width"; Indices_mbdlib "Output Indices"
      mask help: Changes the order of the inputs.
      settings: OpenFcn=|
      | if exist('mbdlib_dialog')
      |    mbdlib_dialog(gcb,'open')
      | else
      |    open_system(gcb, 'mask')
      | end
      settings: CloseFcn=|
      | if exist('mbdlib_selector')
      |    mbdlib_selector(gcb)
      | end
      mask Help: The SELECTOR block is a MULTIPLEXED SELECTOR block, used to change the input/output order of a multiplexed data stream.
      mask Display:
      | port_label('input', 1,'[7]')
      | text(1.0,0.83333,'6', 'horizontalAlignment', 'right')
      | text(1.0,0.5,'7', 'horizontalAlignment', 'right')
      | text(1.0,0.16667,'1', 'horizontalAlignment', 'right')
  column3 : Selector  Tag=MBDLibrary v2007b.1  IndexOptions=Index vector (dialog)  Indices=[2 4 7]  OutputSizes=1  InputPortWidth=7  mask(Mux Selector (MBDLibrary)){InputPortWidth_mbdlib=7, Indices_mbdlib=[2 4 7]}
      mask prompts: InputPortWidth_mbdlib "Input Port Width"; Indices_mbdlib "Output Indices"
      mask help: Changes the order of the inputs.
      settings: OpenFcn=|
      | if exist('mbdlib_dialog')
      |    mbdlib_dialog(gcb,'open')
      | else
      |    open_system(gcb, 'mask')
      | end
      settings: CloseFcn=|
      | if exist('mbdlib_selector')
      |    mbdlib_selector(gcb)
      | end
      mask Help: The SELECTOR block is a MULTIPLEXED SELECTOR block, used to change the input/output order of a multiplexed data stream.
      mask Display:
      | port_label('input', 1,'[7]')
      | text(1.0,0.83333,'2', 'horizontalAlignment', 'right')
      | text(1.0,0.5,'4', 'horizontalAlignment', 'right')
      | text(1.0,0.16667,'7', 'horizontalAlignment', 'right')
  matrixConcat : Concatenate  Tag=MBDLibrary v2007b.1  NumInputs=3  Mode=Multidimensional array  ConcatenateDimension=2  mask(Matrix Concat (MBDLibrary)){concatDim=Horizontal, numInputs_mbdlib=3}
      mask prompts: concatDim "Type of Concatenate"; numInputs_mbdlib "Number of Inputs"
      mask help: Concatenate input signals of the same data type to create a contiguous output signal.
      settings: OpenFcn=|
      | if exist('mbdlib_dialog')
      |    mbdlib_dialog(gcb,'open')
      | else
      |    open_system(gcb, 'mask')
      | end
      settings: CloseFcn=|
      | if exist('mbdlib_matrixConcatenate')
      |    mbdlib_matrixConcatenate(gcb, 'mask')
      | end
      mask Help:
      | The MATRIX CONCAT block concatenates input signals from the dame data type and creates a contigouos output matrix.
      | In vector mode, all input signals must be either vectors or one-row [1xM] matrices or one-column [Mx1] matrices or a combination of vectors and either one-row matrices or one-column matrices. The output is a vector if all inputs are vectors. The output is a one-row or one-column matrix if any of the inputs are one-row or one-column matrices respectively.
      | 
      | Matrix mode treats vector inputs as one-column matrices. The output is always a matrix.
      mask StyleString: popup(Vertical|Horizontal),edit
      mask Display:
      | plot([0.1 0.3 0.3 0.1 0.1], [0.1 0.1 0.9 0.9 0.1])
      | plot([0.4 0.6 0.6 0.4 0.4], [0.1 0.1 0.9 0.9 0.1])
      | plot([0.7 0.9 0.9 0.7 0.7], [0.1 0.1 0.9 0.9 0.1])
  mux : Mux  Tag=MBDLibrary v2007b.1  Inputs=3  mask(Mux (MBDLibrary)){Inputs_mbdlib=3}
      mask prompts: Inputs_mbdlib "Number of Inputs"
      mask help: Converts multipule inputs to a vector.
      settings: OpenFcn=|
      | if exist('mbdlib_dialog')
      |    mbdlib_dialog(gcb,'open')
      | else
      |    open_system(gcb, 'mask')
      | end
      mask Help: The MUX block provides a vector output to the model for separate inputs.  The output order will correspond to the input order (from the first input at the top of the block to the last input at the bottom of the block).
  negative : Gain  Tag=MBDLibrary v2007b.1  Gain=-1  ParameterDataType=fixdt(1,16,0)  ParameterScaling=[]  OutDataType=fixdt(1,16,0)  OutScaling=[]  RndMeth=Zero  mask(Gain (MBDLibrary)){gain_mbdlib=-1}
      mask prompts: gain_mbdlib "Gain"
      mask help: Multiplies the input by the gain.
      settings: OpenFcn=|
      | if exist('mbdlib_dialog')
      |    mbdlib_dialog(gcb,'open')
      | else
      |    open_system(gcb, 'mask')
      | end
      mask Help: The GAIN block multiplies the input by the gain value.  This block may accept any data types other than boolean.  The user must take care to not use a non-integer gain for int32/uint32 inputs.
      mask Display: disp([get_param(gcb, 'Gain') 'x'])
  zero : Constant  Tag=MBDLibrary v2007b.1  Value=0  VectorParams1D=off  OutDataType=fixdt(1,16,0)  OutScaling=[]  mask(Constant (MBDLibrary)){Value_mbdlib=0, OutDataTypeMode_mbdlib=double}
      mask prompts: Value_mbdlib "Constant"; OutDataTypeMode_mbdlib "Data Type"
      mask help: Outputs a constant value
      settings: AttributesFormatString={%<OutDataTypeMode>}
      settings: OpenFcn=|
      | if exist('mbdlib_dialog')
      |    mbdlib_dialog(gcb,'open')
      | else
      |    open_system(gcb, 'mask')
      | end
      settings: CloseFcn=|
      | if exist('mbdlib_dialog')
      |    mbdlib_constant(gcb)
      | end
      mask Help: The CONSTANT block outputs a constant value to the system.
      mask StyleString: edit,popup(double|single|boolean|int32|uint32)
  skewLibOut : Outport  OutDataType=fixdt(1,16,0)  OutScaling=[]
  wires:
  zero/1 -> mux/3
  negative/1 -> mux/2
  column3/1 -> matrixConcat/3
  column2/1 -> matrixConcat/2
  column1/1 -> matrixConcat/1
  matrixConcat/1 -> skewLibOut/1
  mux/1 -> column1/1, column3/1, column2/1
  skewLibIn/1 -> mux/1, negative/1
